simulink model "fuelCycle_w_trapping_multilevel_shutdown"  (R2023b)
settings: Solver=ode15s  StartTime=0.0  StopTime=sim_time  MinStep=5e-5  RelTol=1e-2
values from neighbouring files (symbols this model uses):
  AF = 90    [BOTH_scenario_inputData.m]    (also in FC_scenario_inputData.m; PO_scenario_inputData.m = 0.7; inputData.m = 95; parametric_analysis_AF.m = AF_array(i))
  eta2 = 0.95    [BOTH_scenario_inputData.m]    (also in FC_scenario_inputData.m; PO_scenario_inputData.m; inputData.m; parametric_analysis_eta_tes.m = eta_tes_array(i))
  f51 = 0.33    [BOTH_scenario_inputData.m]    (also in FC_scenario_inputData.m; PO_scenario_inputData.m; inputData.m; worst_case_InputData.m)
  f53 = 0.33    [BOTH_scenario_inputData.m]    (also in FC_scenario_inputData.m; PO_scenario_inputData.m; inputData.m; worst_case_InputData.m)
  f54 = 1 - f51 - f53 - f56    (= 0.3399)    [BOTH_scenario_inputData.m]    (also in FC_scenario_inputData.m; PO_scenario_inputData.m; inputData.m; worst_case_InputData.m)
  f96 = 0.1    [BOTH_scenario_inputData.m]    (also in FC_scenario_inputData.m; PO_scenario_inputData.m; inputData.m; worst_case_InputData.m)
  f_dir = 0.7    [BOTH_scenario_inputData.m]    (also in FC_scenario_inputData.m; PO_scenario_inputData.m = 0.3; inputData.m = 0.3; parametric_analysis_f_dir.m = f_dir_array(i))
  fp3 = 1e-4    (= 0.0001)    [BOTH_scenario_inputData.m]    (also in FC_scenario_inputData.m; PO_scenario_inputData.m; inputData.m; parametric_analysis_f_p.m = f_p(i) / 2)
  fp4 = 1e-4    (= 0.0001)    [BOTH_scenario_inputData.m]    (also in FC_scenario_inputData.m; PO_scenario_inputData.m; inputData.m; parametric_analysis_f_p.m = f_p(i) / 2)
  I_recovered = 0.023 + 0.027 + 0.601    (= 0.651)    [inputData.m]
  I_s_0 = 1.98    [fuelCycleSimulator.m]    (also in parametric_analysis_AF.m = 0.8; parametric_analysis_epsi.m = 0.8; parametric_analysis_eta_tes.m = 0.8; parametric_analysis_f_dir.m = 0.8)
  lambda = 1.73e-9    (= 1.73e-09)    [BOTH_scenario_inputData.m]    (also in FC_scenario_inputData.m; PO_scenario_inputData.m; inputData.m; worst_case_InputData.m)
  N_dot = 8.99e-7    (= 8.99e-07)    [BOTH_scenario_inputData.m]    (also in FC_scenario_inputData.m = 9.3e-07; PO_scenario_inputData.m = 9.3e-07; inputData.m = 9.3e-07; worst_case_InputData.m = 9.3e-07)
  n_trap_tungsten_intrinsic = 2e22/n_tungsten    (= 0.000316284160152)    [inputData_trapping-lap-meschini.m]    (also in inputData_trapping.m = 0.00035)
  n_tungsten_max = [4.75* layer_thickness_induced_traps/FW_thickness, 3.2, 2.5, 6.3]*1e25/n_tungsten    [inputData_trapping-lap-meschini.m]    (also in inputData_trapping.m = [6.9* layer_thickness_induced_traps/FW_thickness, 7, 6, 4.7,)
  Recover_length = 30 * 24 * 8760    (= 6307200)    [inputData.m]
  T1 = 1/((1 + epsi)/tau1 + lambda)    [BOTH_scenario_inputData.m]    (also in FC_scenario_inputData.m; PO_scenario_inputData.m; inputData.m; parametric_analysis_epsi.m)
  T12 = 1/((1 + epsi)/tau12 + lambda)    [BOTH_scenario_inputData.m]    (also in FC_scenario_inputData.m; PO_scenario_inputData.m; inputData.m; parametric_analysis_epsi.m)
  T2 = 1/((1 + epsi)/tau2 + lambda)    [BOTH_scenario_inputData.m]    (also in FC_scenario_inputData.m; PO_scenario_inputData.m; inputData.m; parametric_analysis_epsi.m)
  T3 = 1/((1 + 0)/tau3 + lambda)    [BOTH_scenario_inputData.m]    (also in FC_scenario_inputData.m; PO_scenario_inputData.m; inputData.m; parametric_analysis_epsi.m)
  T4 = 1/((1 + 0)/tau4 + lambda)    [BOTH_scenario_inputData.m]    (also in FC_scenario_inputData.m; PO_scenario_inputData.m; inputData.m; parametric_analysis_epsi.m)
  T7 = 1/((1 + epsi)/tau7 + lambda)    [BOTH_scenario_inputData.m]    (also in FC_scenario_inputData.m; PO_scenario_inputData.m; inputData.m; parametric_analysis_epsi.m)
  T8 = 1/((1 + epsi)/tau8 + lambda)    [BOTH_scenario_inputData.m]    (also in FC_scenario_inputData.m; PO_scenario_inputData.m; inputData.m; parametric_analysis_TBE.m)
  T9 = 1/((1 + epsi)/tau9 + lambda)    [BOTH_scenario_inputData.m]    (also in FC_scenario_inputData.m; PO_scenario_inputData.m; inputData.m; parametric_analysis_TBE.m)
  tau1 = 1.25*3600    (= 4500)    [BOTH_scenario_inputData.m]    (also in FC_scenario_inputData.m; PO_scenario_inputData.m; inputData.m; parametric_analysis_t_blanket.m = tau1_array(i))
  tau12 = 100    [BOTH_scenario_inputData.m]    (also in FC_scenario_inputData.m; PO_scenario_inputData.m; inputData.m; worst_case_InputData.m)
  tau2 = 1*24*3600    (= 86400)    [BOTH_scenario_inputData.m]    (also in FC_scenario_inputData.m; PO_scenario_inputData.m; inputData.m; worst_case_InputData.m)
  tau3 = 1000    [BOTH_scenario_inputData.m]    (also in FC_scenario_inputData.m; PO_scenario_inputData.m; inputData.m; worst_case_InputData.m)
  tau4 = 1000    [BOTH_scenario_inputData.m]    (also in FC_scenario_inputData.m; PO_scenario_inputData.m; inputData.m; worst_case_InputData.m)
  tau5 = 1000    [BOTH_scenario_inputData.m]    (also in FC_scenario_inputData.m; PO_scenario_inputData.m; inputData.m; worst_case_InputData.m)
  tau6 = 3600    [BOTH_scenario_inputData.m]    (also in FC_scenario_inputData.m; PO_scenario_inputData.m; inputData.m; worst_case_InputData.m)
  tau7 = 600    [BOTH_scenario_inputData.m]    (also in FC_scenario_inputData.m; PO_scenario_inputData.m; inputData.m; worst_case_InputData.m)
  tau8 = 0.1*3600    (= 360)    [BOTH_scenario_inputData.m]    (also in FC_scenario_inputData.m; PO_scenario_inputData.m; inputData.m = 3600; parametric_analysis_TBE.m = t_p*0.1)
  tau9 = 0.9*3600    (= 3240)    [BOTH_scenario_inputData.m]    (also in FC_scenario_inputData.m; PO_scenario_inputData.m = 14040; inputData.m = 10800; parametric_analysis_TBE.m = t_p*0.9)
  TBE = 0.1    [BOTH_scenario_inputData.m]    (also in FC_scenario_inputData.m = 0.02; PO_scenario_inputData.m; inputData.m = 0.02; parametric_analysis_AF.m = TBE_array(j))
  TBR = 1.115    [fuelCycleSimulator.m]    (also in parametric_analysis_AF.m = 1; parametric_analysis_TBE.m = 1; parametric_analysis_epsi.m = 1; parametric_analysis_eta_tes.m = 1)
  trap_creation_factor_W = [1* layer_thickness_induced_traps/FW_thickness, 0.9, 0.6, 1]*1e28/n_tungsten    [inputData_trapping-lap-meschini.m]    (also in inputData_trapping.m = [9* layer_thickness_induced_traps/FW_thickness, 4.2, 2.5, 5,)
libraries: arc x23, arc_2 x11
settings Model: SimulationMode=accelerator  Creator=smesc  LastModifiedBy=meschini
settings SolverCC: InitialStep=5e-5  MaxConsecutiveMinStep=100000  ShapePreserveControl=EnableAll  ZeroCrossAlgorithm=Adaptive  SolverResetMethod=Robust
settings OptimizationCC: ReuseModelBlockBuffer=off
settings HardwareCC: ProdBitPerPointer=32  ProdBitPerSizeT=32  ProdBitPerPtrDiffT=32  ProdWordSize=32  ProdHWDeviceType=Intel->x86-32 (Windows32)
settings ModelReferenceCC: EnableRefExpFcnMdlSchedulingChecks=on

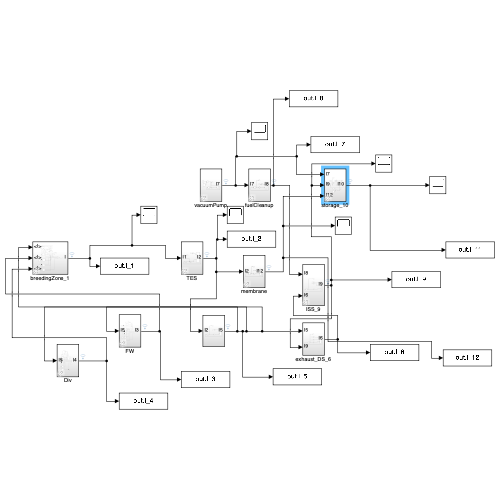
[thumbnail: Simulink's stored preview of the top-level diagram]
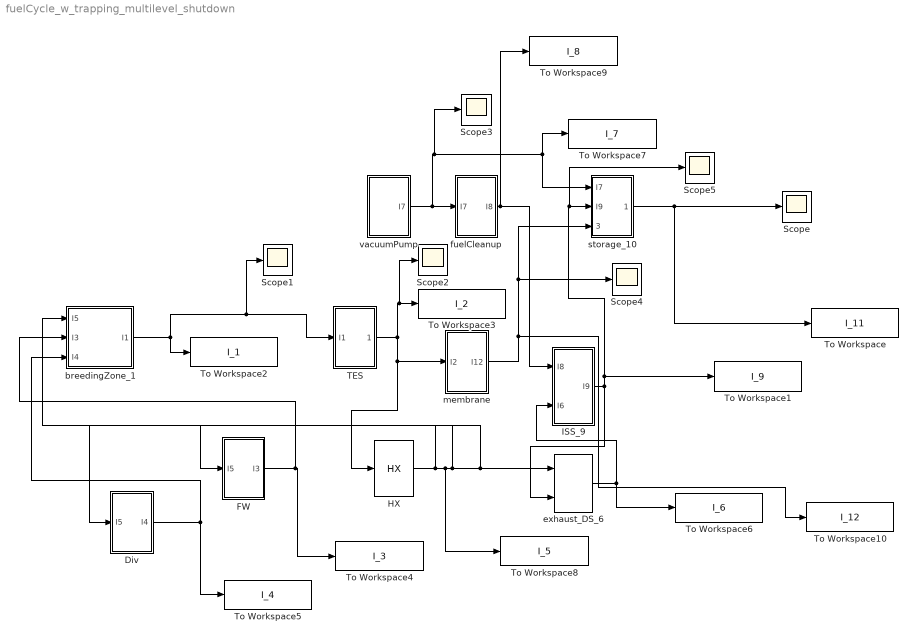
== system fuelCycle_w_trapping_multilevel_shutdown ==
  Div : Subsystem  AncestorBlock=arc/divertor_4
      settings: LibrarySourceBlock=arc/divertor_4
  FW : Subsystem  AncestorBlock=arc/FW_3
      settings: LibrarySourceBlock=arc/FW_3
  HX : arc/HX  Tag=HX  SystemSampleTime=-1  VariantActivationTime=update diagram  AllowFlexibleInterface=on  Latency=0  AutoFrameSizeCalculation=off
  ISS_9 : Subsystem  AncestorBlock=arc/ISS_9
      settings: LibrarySourceBlock=arc/ISS_9
  Scope{,1..5} (6 alike) : Scope
  TES : Subsystem  AncestorBlock=arc/TES_2
      settings: LibrarySourceBlock=arc/TES_2
  To Workspace : ToWorkspace  VariableName=I_11  SampleTime=-1
  To Workspace1 : ToWorkspace  VariableName=I_9  SampleTime=-1
  To Workspace10 : ToWorkspace  VariableName=I_12  SampleTime=-1
  To Workspace2 : ToWorkspace  VariableName=I_1  SampleTime=-1
  To Workspace3 : ToWorkspace  VariableName=I_2  SampleTime=-1
  To Workspace4 : ToWorkspace  VariableName=I_3  SampleTime=-1
  To Workspace5 : ToWorkspace  VariableName=I_4  SampleTime=-1
  To Workspace6 : ToWorkspace  VariableName=I_6  SampleTime=-1
  To Workspace7 : ToWorkspace  VariableName=I_7  SampleTime=-1
  To Workspace8 : ToWorkspace  VariableName=I_5  SampleTime=-1
  To Workspace9 : ToWorkspace  VariableName=I_8  SampleTime=-1
  breedingZone_1 : Subsystem  AncestorBlock=arc/breedingZone_1
      settings: LibrarySourceBlock=arc/breedingZone_1
  exhaust_DS_6 : arc/exhaust_DS  SystemSampleTime=-1  VariantActivationTime=update diagram  AllowFlexibleInterface=on  Latency=0  AutoFrameSizeCalculation=off
      link override Gain: Gain=f56/tau5
  fuelCleanup : Subsystem  AncestorBlock=arc/fuelCleanUp
  membrane : Subsystem  AncestorBlock=arc/fuelCleanUp_8
      settings: LibrarySourceBlock=arc/fuelCleanUp_8
  storage_10 : Subsystem  AncestorBlock=arc/storage_10
      settings: LibrarySourceBlock=arc/storage_10
  vacuumPump : Subsystem  AncestorBlock=arc/pump_7
      settings: LibrarySourceBlock=arc/pump_7
  wires:
  breedingZone_1/1(I1) -> Scope1/1, TES/1(I1), To Workspace2/1
  storage_10/1(I10) -> To Workspace/1, Scope/1
  FW/1(I3) -> breedingZone_1/2(I3), To Workspace4/1
  Div/1(I4) -> breedingZone_1/3(I4), To Workspace5/1
  membrane/1(I12) -> To Workspace10/1, Scope4/1, storage_10/3(I12)
  fuelCleanup/1(I8) -> To Workspace9/1, ISS_9/1(I8)
  vacuumPump/1(I7) -> Scope3/1, To Workspace7/1, storage_10/1(I7), fuelCleanup/1(I7)
  exhaust_DS_6/1 -> ISS_9/2(I6), To Workspace6/1
  ISS_9/1(I9) -> exhaust_DS_6/2, Scope5/1, storage_10/2(I9), To Workspace1/1
  HX/1 -> FW/1(I5), To Workspace8/1, Div/1(I5), exhaust_DS_6/1, breedingZone_1/1(I5)
  TES/1(Output) -> Scope2/1, To Workspace3/1, membrane/1(I2), HX/1

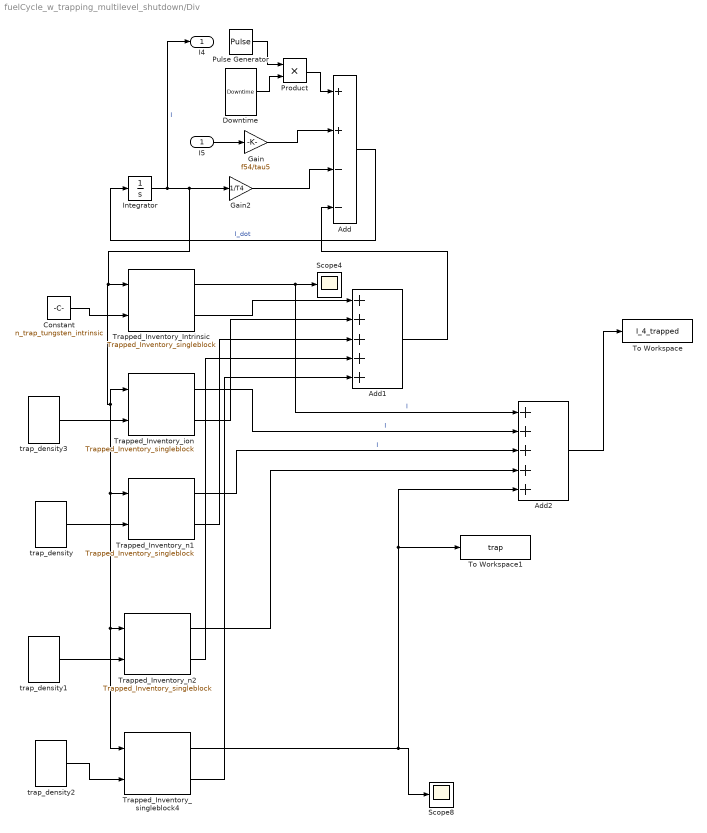
== system fuelCycle_w_trapping_multilevel_shutdown/Div ==
  I5 : Inport
  Add : Sum  Inputs=++--
  Add1 : Sum  Inputs=+++++
  Add2 : Sum  Inputs=+++++
  Constant : Constant  Value=n_trap_tungsten_intrinsic
  Downtime : arc/Downtime  T_shutdown=T_replacement  T_restart=T_restart
  Gain : Gain  Gain=f54/tau5
  Gain2 : Gain  Gain=1/T4
  Integrator : Integrator
  Product : Product
  Pulse Generator : DiscretePulseGenerator  PulseType=Time based  Amplitude=fp4*N_dot/TBE  Period=1800  PulseWidth=AF
  Scope4 : Scope
  Scope8 : Scope
  To Workspace : ToWorkspace  VariableName=I_4_trapped  SampleTime=-1
  To Workspace1 : ToWorkspace  VariableName=trap  SampleTime=-1
  Trapped_Inventory_Intrinsic : arc/Trapped_Inventory_singleblock  SystemSampleTime=-1  VariantActivationTime=update diagram  AllowFlexibleInterface=on  Latency=0  AutoFrameSizeCalculation=off
      link override Trap_detrap_ml2: n_trap=n_trap_tungsten(1)  tau_trap=tau_trap_tungsten  tau_detrap=tau_detrap_tungsten(1)  PM_host=PM_tungsten  M_host=M_tungsten  n_solute=n_solute_tungsten
  Trapped_Inventory_ion : arc/Trapped_Inventory_singleblock  SystemSampleTime=-1  VariantActivationTime=update diagram  AllowFlexibleInterface=on  Latency=0  AutoFrameSizeCalculation=off
      link override Trap_detrap_ml2: n_trap=n_trap_tungsten(2)  tau_trap=tau_trap_tungsten  tau_detrap=tau_detrap_tungsten(2)  PM_host=PM_tungsten  M_host=M_tungsten  n_solute=n_solute_tungsten
  Trapped_Inventory_n1 : arc/Trapped_Inventory_singleblock  SystemSampleTime=-1  VariantActivationTime=update diagram  AllowFlexibleInterface=on  Latency=0  AutoFrameSizeCalculation=off
      link override Trap_detrap_ml2: n_trap=n_trap_tungsten(3)  tau_trap=tau_trap_tungsten  tau_detrap=tau_detrap_tungsten(3)  PM_host=PM_tungsten  M_host=M_tungsten  n_solute=n_solute_tungsten
  Trapped_Inventory_n2 : arc/Trapped_Inventory_singleblock  SystemSampleTime=-1  VariantActivationTime=update diagram  AllowFlexibleInterface=on  Latency=0  AutoFrameSizeCalculation=off
      link override Trap_detrap_ml2: n_trap=n_trap_tungsten(4)  tau_trap=tau_trap_tungsten  tau_detrap=tau_detrap_tungsten(4)  PM_host=PM_tungsten  M_host=M_tungsten  n_solute=n_solute_tungsten
  Trapped_Inventory_singleblock4 : arc/Trapped_Inventory_singleblock  SystemSampleTime=-1  VariantActivationTime=update diagram  AllowFlexibleInterface=on  Latency=0  AutoFrameSizeCalculation=off
      link override Trap_detrap_ml2: n_trap=n_trap_tungsten(5)  tau_trap=tau_trap_tungsten  tau_detrap=tau_detrap_tungsten(5)  PM_host=PM_tungsten  M_host=M_tungsten  n_solute=n_solute_tungsten
  trap_density : arc_2/trap_density  n_max=n_tungsten_max(2)  damage_rate=damage_rate  trap_creation_factor=trap_creation_factor_W(2)  A_0=A_0  E_annealing=E_annealing  T_material=T_tungsten
  trap_density1 : arc_2/trap_density  n_max=n_tungsten_max(3)  damage_rate=damage_rate  trap_creation_factor=trap_creation_factor_W(3)  A_0=A_0  E_annealing=E_annealing  T_material=T_tungsten
  trap_density2 : arc_2/trap_density  n_max=n_tungsten_max(4)  damage_rate=damage_rate  trap_creation_factor=trap_creation_factor_W(4)  A_0=A_0  E_annealing=E_annealing  T_material=T_tungsten
  trap_density3 : arc_2/trap_density  n_max=n_tungsten_max(1)  damage_rate=damage_rate  trap_creation_factor=trap_creation_factor_W(1)  A_0=A_0  E_annealing=E_annealing  T_material=T_tungsten
  I4 : Outport
  wires:
  Gain/1 -> Add/2
  Add/1 -> Integrator/1  "I_dot"
  Gain2/1 -> Add/3
  I5/1 -> Gain/1
  Integrator/1 -> Trapped_Inventory_ion/1, Trapped_Inventory_n1/1, Trapped_Inventory_singleblock4/1, Trapped_Inventory_n2/1, Trapped_Inventory_Intrinsic/1, Gain2/1, I4/1  "I"
  Trapped_Inventory_n1/1 -> Add2/3  "I"
  trap_density2/1 -> Trapped_Inventory_singleblock4/2
  Trapped_Inventory_ion/1 -> Add2/2  "I"
  Add1/1 -> Add/4
  trap_density/1 -> Trapped_Inventory_n1/2
  Trapped_Inventory_ion/2 -> Add1/2
  Trapped_Inventory_Intrinsic/1 -> Add2/1, Scope4/1  "I"
  Add2/1 -> To Workspace/1
  Trapped_Inventory_n2/1 -> Add2/4
  Trapped_Inventory_Intrinsic/2 -> Add1/1
  trap_density1/1 -> Trapped_Inventory_n2/2
  trap_density3/1 -> Trapped_Inventory_ion/2
  Constant/1 -> Trapped_Inventory_Intrinsic/2
  Trapped_Inventory_n1/2 -> Add1/3
  Trapped_Inventory_n2/2 -> Add1/4
  Trapped_Inventory_singleblock4/1 -> Scope8/1, To Workspace1/1, Add2/5
  Trapped_Inventory_singleblock4/2 -> Add1/5
  Pulse Generator/1 -> Product/1
  Downtime/1 -> Product/2
  Product/1 -> Add/1

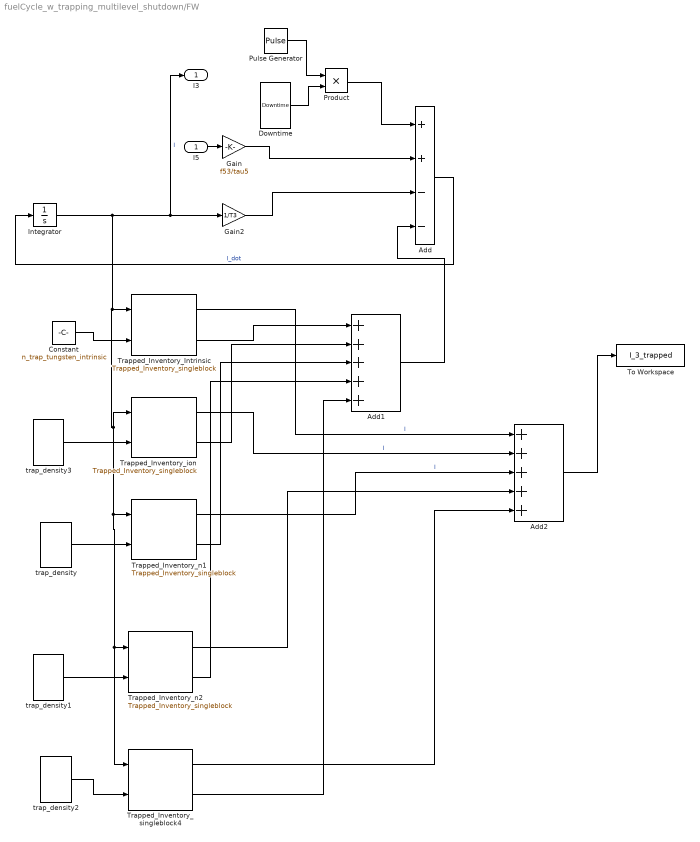
== system fuelCycle_w_trapping_multilevel_shutdown/FW ==
  I5 : Inport
  Add : Sum  Inputs=++--
  Add1 : Sum  Inputs=+++++
  Add2 : Sum  Inputs=+++++
  Constant : Constant  Value=n_trap_tungsten_intrinsic
  Downtime : arc/Downtime  T_shutdown=T_replacement  T_restart=T_restart
  Gain : Gain  Gain=f53/tau5
  Gain2 : Gain  Gain=1/T3
  Integrator : Integrator
  Product : Product
  Pulse Generator : DiscretePulseGenerator  PulseType=Time based  Amplitude=fp3*N_dot/TBE  Period=1800  PulseWidth=AF
  To Workspace : ToWorkspace  VariableName=I_3_trapped  SampleTime=-1
  Trapped_Inventory_Intrinsic : arc/Trapped_Inventory_singleblock  SystemSampleTime=-1  VariantActivationTime=update diagram  AllowFlexibleInterface=on  Latency=0  AutoFrameSizeCalculation=off
      link override Trap_detrap_ml2: n_trap=n_trap_tungsten(1)  tau_trap=tau_trap_tungsten  tau_detrap=tau_detrap_tungsten(1)  PM_host=PM_tungsten  M_host=M_tungsten  n_solute=n_solute_tungsten
  Trapped_Inventory_ion : arc/Trapped_Inventory_singleblock  SystemSampleTime=-1  VariantActivationTime=update diagram  AllowFlexibleInterface=on  Latency=0  AutoFrameSizeCalculation=off
      link override Trap_detrap_ml2: n_trap=n_trap_tungsten(2)  tau_trap=tau_trap_tungsten  tau_detrap=tau_detrap_tungsten(2)  PM_host=PM_tungsten  M_host=M_tungsten  n_solute=n_solute_tungsten
  Trapped_Inventory_n1 : arc/Trapped_Inventory_singleblock  SystemSampleTime=-1  VariantActivationTime=update diagram  AllowFlexibleInterface=on  Latency=0  AutoFrameSizeCalculation=off
      link override Trap_detrap_ml2: n_trap=n_trap_tungsten(3)  tau_trap=tau_trap_tungsten  tau_detrap=tau_detrap_tungsten(3)  PM_host=PM_tungsten  M_host=M_tungsten  n_solute=n_solute_tungsten
  Trapped_Inventory_n2 : arc/Trapped_Inventory_singleblock  SystemSampleTime=-1  VariantActivationTime=update diagram  AllowFlexibleInterface=on  Latency=0  AutoFrameSizeCalculation=off
      link override Trap_detrap_ml2: n_trap=n_trap_tungsten(4)  tau_trap=tau_trap_tungsten  tau_detrap=tau_detrap_tungsten(4)  PM_host=PM_tungsten  M_host=M_tungsten  n_solute=n_solute_tungsten
  Trapped_Inventory_singleblock4 : arc/Trapped_Inventory_singleblock  SystemSampleTime=-1  VariantActivationTime=update diagram  AllowFlexibleInterface=on  Latency=0  AutoFrameSizeCalculation=off
      link override Trap_detrap_ml2: n_trap=n_trap_tungsten(5)  tau_trap=tau_trap_tungsten  tau_detrap=tau_detrap_tungsten(5)  PM_host=PM_tungsten  M_host=M_tungsten  n_solute=n_solute_tungsten
  trap_density : arc_2/trap_density  n_max=n_tungsten_max(2)  damage_rate=damage_rate  trap_creation_factor=trap_creation_factor_W(2)  A_0=A_0  E_annealing=E_annealing  T_material=T_tungsten
  trap_density1 : arc_2/trap_density  n_max=n_tungsten_max(3)  damage_rate=damage_rate  trap_creation_factor=trap_creation_factor_W(3)  A_0=A_0  E_annealing=E_annealing  T_material=T_tungsten
  trap_density2 : arc_2/trap_density  n_max=n_tungsten_max(4)  damage_rate=damage_rate  trap_creation_factor=trap_creation_factor_W(4)  A_0=A_0  E_annealing=E_annealing  T_material=T_tungsten
  trap_density3 : arc_2/trap_density  n_max=n_tungsten_max(1)  damage_rate=damage_rate  trap_creation_factor=trap_creation_factor_W(1)  A_0=A_0  E_annealing=E_annealing  T_material=T_tungsten
  I3 : Outport
  wires:
  Gain2/1 -> Add/3
  Add/1 -> Integrator/1  "I_dot"
  Gain/1 -> Add/2
  I5/1 -> Gain/1
  trap_density1/1 -> Trapped_Inventory_n2/2
  Constant/1 -> Trapped_Inventory_Intrinsic/2
  Trapped_Inventory_Intrinsic/2 -> Add1/1
  Trapped_Inventory_Intrinsic/1 -> Add2/1  "I"
  Trapped_Inventory_ion/2 -> Add1/2
  trap_density/1 -> Trapped_Inventory_n1/2
  Add2/1 -> To Workspace/1
  Add1/1 -> Add/4
  Integrator/1 -> Trapped_Inventory_ion/1, Trapped_Inventory_n1/1, Trapped_Inventory_singleblock4/1, Trapped_Inventory_n2/1, Trapped_Inventory_Intrinsic/1, I3/1, Gain2/1  "I"
  Trapped_Inventory_ion/1 -> Add2/2  "I"
  trap_density2/1 -> Trapped_Inventory_singleblock4/2
  trap_density3/1 -> Trapped_Inventory_ion/2
  Trapped_Inventory_n1/1 -> Add2/3  "I"
  Trapped_Inventory_n1/2 -> Add1/3
  Trapped_Inventory_n2/1 -> Add2/4
  Trapped_Inventory_singleblock4/1 -> Add2/5
  Trapped_Inventory_singleblock4/2 -> Add1/5
  Trapped_Inventory_n2/2 -> Add1/4
  Pulse Generator/1 -> Product/1
  Downtime/1 -> Product/2
  Product/1 -> Add/1

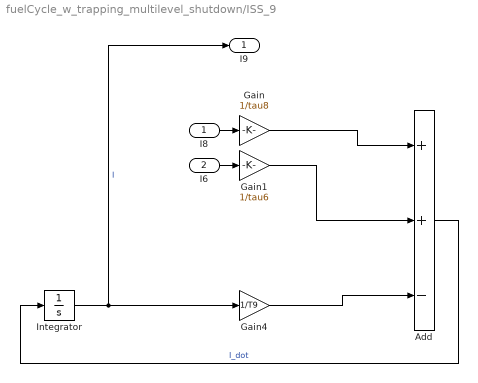
== system fuelCycle_w_trapping_multilevel_shutdown/ISS_9 ==
  I8 : Inport
  I6 : Inport  Port=2
  Add : Sum  Inputs=++-
  Gain : Gain  Gain=1/tau8
  Gain1 : Gain  Gain=1/tau6
  Gain4 : Gain  Gain=1/T9
  Integrator : Integrator
  I9 : Outport
  wires:
  I8/1 -> Gain/1
  Gain1/1 -> Add/2
  I6/1 -> Gain1/1
  Add/1 -> Integrator/1  "I_dot"
  Integrator/1 -> Gain4/1, I9/1  "I"
  Gain/1 -> Add/1
  Gain4/1 -> Add/3

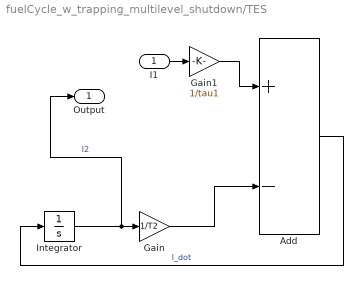
== system fuelCycle_w_trapping_multilevel_shutdown/TES ==
  I1 : Inport
  Add : Sum  Inputs=+-
  Gain : Gain  Gain=1/T2
  Gain1 : Gain  Gain=1/tau1
  Integrator : Integrator
  Output : Outport
  wires:
  Gain/1 -> Add/2
  I1/1 -> Gain1/1
  Gain1/1 -> Add/1
  Integrator/1 -> Gain/1, Output/1  "I2"
  Add/1 -> Integrator/1  "I_dot"

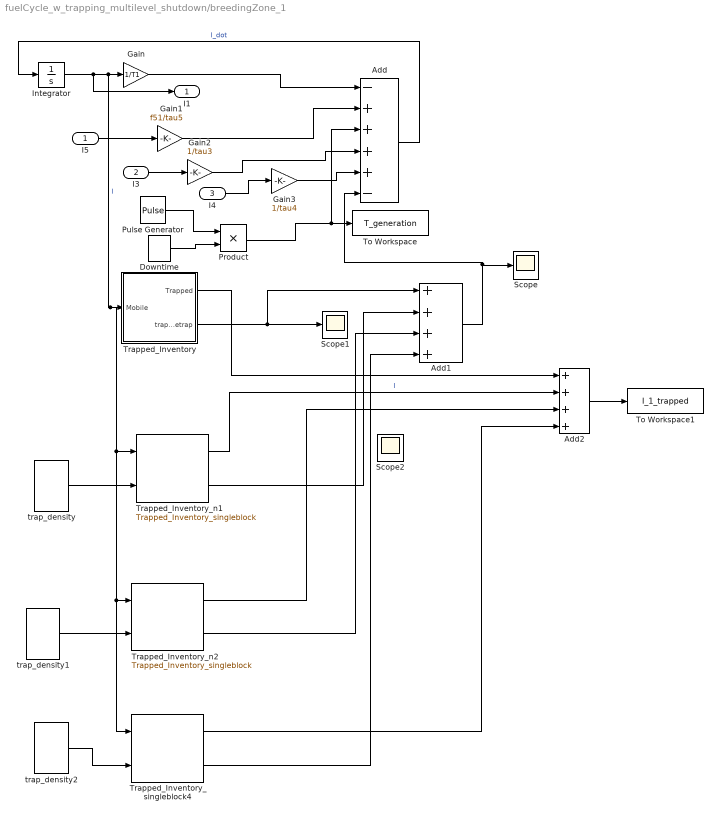
== system fuelCycle_w_trapping_multilevel_shutdown/breedingZone_1 ==
  I5 : Inport
  I3 : Inport  Port=2
  I4 : Inport  Port=3
  Add : Sum  Inputs=-++++-
  Add1 : Sum  Inputs=++++
  Add2 : Sum  Inputs=++++
  Downtime : arc/Downtime  T_shutdown=T_replacement  T_restart=T_restart
  Gain : Gain  Gain=1/T1
  Gain1 : Gain  Gain=f51/tau5
  Gain2 : Gain  Gain=1/tau3
  Gain3 : Gain  Gain=1/tau4
  Integrator : Integrator
  Product : Product
  Pulse Generator : DiscretePulseGenerator  PulseType=Time based  Amplitude=N_dot * TBR  Period=1800  PulseWidth=AF
  Scope : Scope
  Scope1 : Scope
  Scope2 : Scope
  To Workspace : ToWorkspace  VariableName=T_generation  SaveFormat=Timeseries  SampleTime=-1
  To Workspace1 : ToWorkspace  VariableName=I_1_trapped  SampleTime=-1
  Trapped_Inventory : Subsystem
  Trapped_Inventory_n1 : arc/Trapped_Inventory_singleblock  SystemSampleTime=-1  VariantActivationTime=update diagram  AllowFlexibleInterface=on  Latency=0  AutoFrameSizeCalculation=off
      link override Trap_detrap_ml2: n_trap=n_trap_tungsten(3)  tau_trap=tau_trap_structural  tau_detrap=tau_detrap_tungsten(3)  PM_host=PM_structural  M_host=M_structural  n_solute=n_solute_structural
  Trapped_Inventory_n2 : arc/Trapped_Inventory_singleblock  SystemSampleTime=-1  VariantActivationTime=update diagram  AllowFlexibleInterface=on  Latency=0  AutoFrameSizeCalculation=off
      link override Trap_detrap_ml2: n_trap=n_trap_tungsten(4)  tau_trap=tau_trap_structural  tau_detrap=tau_detrap_tungsten(4)  PM_host=PM_structural  M_host=M_structural  n_solute=n_solute_structural
  Trapped_Inventory_singleblock4 : arc/Trapped_Inventory_singleblock  SystemSampleTime=-1  VariantActivationTime=update diagram  AllowFlexibleInterface=on  Latency=0  AutoFrameSizeCalculation=off
      link override Trap_detrap_ml2: n_trap=n_trap_tungsten(5)  tau_trap=tau_detrap_structural  tau_detrap=tau_detrap_tungsten(5)  PM_host=PM_structural  M_host=M_structural  n_solute=n_solute_structural
  trap_density : arc_2/trap_density  n_max=n_tungsten_max(2)  damage_rate=damage_rate  trap_creation_factor=trap_creation_factor_W(2)  A_0=A_0  E_annealing=E_annealing  T_material=T_structural
  trap_density1 : arc_2/trap_density  n_max=n_tungsten_max(3)  damage_rate=damage_rate  trap_creation_factor=trap_creation_factor_W(3)  A_0=A_0  E_annealing=E_annealing  T_material=T_structural
  trap_density2 : arc_2/trap_density  n_max=n_tungsten_max(4)  damage_rate=damage_rate  trap_creation_factor=trap_creation_factor_W(4)  A_0=A_0  E_annealing=E_annealing  T_material=T_structural
  I1 : Outport
  wires:
  Add/1 -> Integrator/1  "I_dot"
  Gain1/1 -> Add/2
  Gain/1 -> Add/1
  I5/1 -> Gain1/1
  I3/1 -> Gain2/1
  Gain2/1 -> Add/4
  I4/1 -> Gain3/1
  Gain3/1 -> Add/5
  Trapped_Inventory/1(Trapped) -> Add2/1
  Add1/1 -> Scope/1, Add/6
  Add2/1 -> To Workspace1/1
  Trapped_Inventory_n1/1 -> Add2/2  "I"
  Trapped_Inventory/2(trap_detrap) -> Add1/1, Scope1/1
  trap_density2/1 -> Trapped_Inventory_singleblock4/2
  Integrator/1 -> Trapped_Inventory_n1/1, Trapped_Inventory_singleblock4/1, Trapped_Inventory_n2/1, Trapped_Inventory/1(Mobile), Gain/1, I1/1  "I"
  trap_density1/1 -> Trapped_Inventory_n2/2
  trap_density/1 -> Trapped_Inventory_n1/2
  Trapped_Inventory_n2/1 -> Add2/3
  Trapped_Inventory_singleblock4/1 -> Add2/4
  Trapped_Inventory_singleblock4/2 -> Add1/4
  Trapped_Inventory_n2/2 -> Add1/3
  Trapped_Inventory_n1/2 -> Add1/2
  Pulse Generator/1 -> Product/1
  Downtime/1 -> Product/2
  Product/1 -> To Workspace/1, Add/3

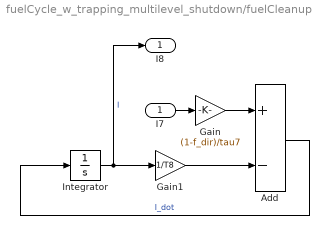
== system fuelCycle_w_trapping_multilevel_shutdown/fuelCleanup ==
  I7 : Inport
  Add : Sum  Inputs=+-
  Gain : Gain  Gain=(1-f_dir)/tau7
  Gain1 : Gain  Gain=1/T8
  Integrator : Integrator
  I8 : Outport
  wires:
  I7/1 -> Gain/1
  Gain1/1 -> Add/2
  Add/1 -> Integrator/1  "I_dot"
  Integrator/1 -> Gain1/1, I8/1  "I"
  Gain/1 -> Add/1

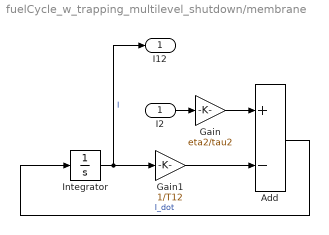
== system fuelCycle_w_trapping_multilevel_shutdown/membrane ==
  I2 : Inport
  Add : Sum  Inputs=+-
  Gain : Gain  Gain=eta2/tau2
  Gain1 : Gain  Gain=1/T12
  Integrator : Integrator
  I12 : Outport
  wires:
  I2/1 -> Gain/1
  Gain1/1 -> Add/2
  Add/1 -> Integrator/1  "I_dot"
  Integrator/1 -> Gain1/1, I12/1  "I"
  Gain/1 -> Add/1

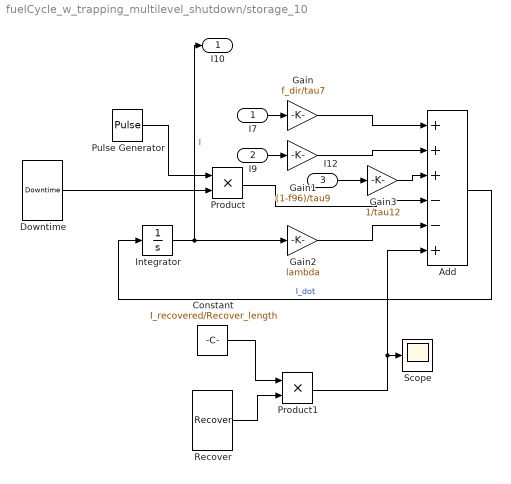
== system fuelCycle_w_trapping_multilevel_shutdown/storage_10 ==
  I7 : Inport
  I9 : Inport  Port=2
  I12 : Inport  Port=3
  Add : Sum  Inputs=+++--+
  Constant : Constant  Value=I_recovered/Recover_length
  Downtime : arc/Downtime  T_shutdown=T_replacement  T_restart=T_restart
  Gain : Gain  Gain=f_dir/tau7
  Gain1 : Gain  Gain=(1-f96)/tau9
  Gain2 : Gain  Gain=lambda
  Gain3 : Gain  Gain=1/tau12
  Integrator : Integrator  InitialCondition=I_s_0
  Product : Product
  Product1 : Product
  Pulse Generator : DiscretePulseGenerator  PulseType=Time based  Amplitude=N_dot/TBE  Period=1800  PulseWidth=AF
  Recover : arc/Recover  T_recover_start=T_recover_start  T_recover_stop=T_recover_stop
  Scope : Scope
  I10 : Outport
  wires:
  Integrator/1 -> Gain2/1, I10/1  "I"
  I9/1 -> Gain1/1
  Gain2/1 -> Add/5
  I7/1 -> Gain/1
  Gain1/1 -> Add/2
  Gain/1 -> Add/1
  I12/1 -> Gain3/1
  Gain3/1 -> Add/3
  Add/1 -> Integrator/1  "I_dot"
  Pulse Generator/1 -> Product/1
  Downtime/1 -> Product/2
  Product/1 -> Add/4
  Constant/1 -> Product1/1
  Product1/1 -> Add/6, Scope/1
  Recover/1 -> Product1/2

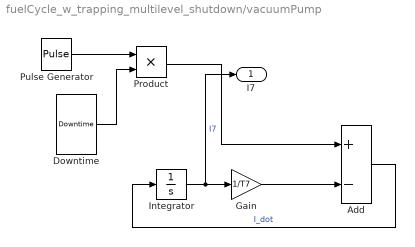
== system fuelCycle_w_trapping_multilevel_shutdown/vacuumPump ==
  Add : Sum  Inputs=+-
  Downtime : arc/Downtime  T_shutdown=T_replacement  T_restart=T_restart
  Gain : Gain  Gain=1/T7
  Integrator : Integrator
  Product : Product
  Pulse Generator : DiscretePulseGenerator  PulseType=Time based  Amplitude=(1-TBE-fp3-fp4)*N_dot/TBE  Period=1800  PulseWidth=AF
  I7 : Outport
  wires:
  Gain/1 -> Add/2
  Integrator/1 -> Gain/1, I7/1  "I7"
  Add/1 -> Integrator/1  "I_dot"
  Pulse Generator/1 -> Product/1
  Downtime/1 -> Product/2
  Product/1 -> Add/1

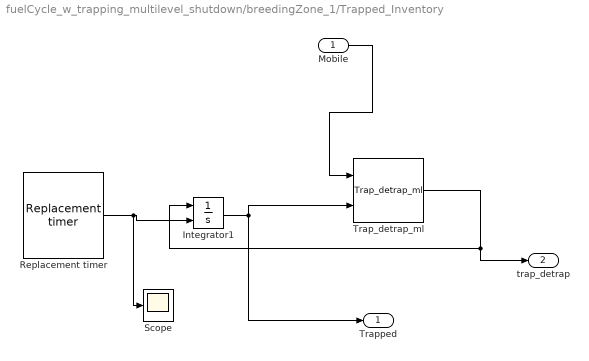
== system fuelCycle_w_trapping_multilevel_shutdown/breedingZone_1/Trapped_Inventory ==
  Mobile : Inport
  Integrator1 : Integrator  ExternalReset=falling
  Replacement timer : arc/Replacement timer  T_replacement=T_replacement
  Scope : Scope
  Trap_detrap_ml : arc/Trap_detrap_ml  n_trap=n_trap_structural  tau_trap=tau_trap_structural  tau_detrap=tau_detrap_structural  n_solute=n_solute_structural  PM_host=PM_structural  PM_tritium=PM_tritium  M_host=M_structural
  Trapped : Outport
  trap_detrap : Outport  Port=2
  wires:
  Mobile/1 -> Trap_detrap_ml/1
  Integrator1/1 -> Trap_detrap_ml/2, Trapped/1
  Trap_detrap_ml/1 -> trap_detrap/1, Integrator1/1
  Replacement timer/1 -> Scope/1, Integrator1/2
